simulink model "trajetorianominal2Simulink"  (R2019a)
settings: Solver=VariableStepAuto  StartTime=0.0  StopTime=170  RelTol=1e-3
undefined symbols (not defined in the file): A, B, C
settings Model: Creator=Cliente  LastModifiedBy=Cliente

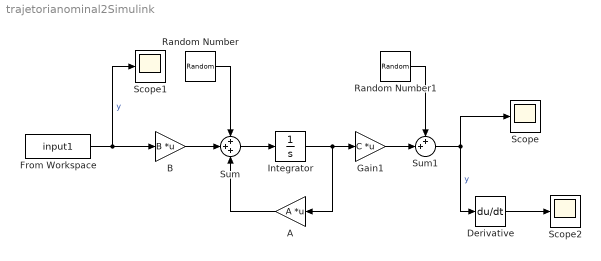
== system trajetorianominal2Simulink ==
  A : Gain  Gain=A  Multiplication=Matrix(K*u) (u vector)
  B : Gain  Gain=B  Multiplication=Matrix(K*u)
  Derivative : Derivative
  From Workspace : FromWorkspace  VariableName=input1  SampleTime=0
  Gain1 : Gain  Gain=C  Multiplication=Matrix(K*u) (u vector)
  Integrator : Integrator  InitialCondition=[0;0]
  Random Number : RandomNumber  Variance=1.5  SampleTime=0.05
  Random Number1 : RandomNumber  Variance=1.031  SampleTime=0.1
  Scope : Scope
  Scope1 : Scope
  Scope2 : Scope
  Sum : Sum  Inputs=+++
  Sum1 : Sum  Inputs=++|
  wires:
  Integrator/1 -> A/1, Gain1/1
  A/1 -> Sum/3
  Sum/1 -> Integrator/1
  Derivative/1 -> Scope2/1
  B/1 -> Sum/2
  From Workspace/1 -> Scope1/1, B/1  "y"
  Random Number/1 -> Sum/1
  Sum1/1 -> Scope/1, Derivative/1  "y"
  Gain1/1 -> Sum1/2
  Random Number1/1 -> Sum1/1
